simulink model "selector4"  (R2015a)
settings: Solver=FixedStepDiscrete  StartTime=0.0  StopTime=10.0  RelTol=1e-3
settings Model: CovSFcnEnable=off  Creator=arnaud  LastModifiedBy=ktrinh
settings DataIOCC: SaveFormat=StructureWithTime  SignalLoggingSaveFormat=ModelDataLogs
settings OptimizationCC: ExpressionDepthLimit=2147483647
settings DebuggingCC: UnderspecifiedInitializationDetection=Classic  MergeDetectMultiDrivingBlocksExec=none  SolverPrmCheckMsg=warning  FcnCallInpInsideContextMsg=EnableAllAsWarning  StateNameClashWarn=warning
settings GRTTargetCC: CombineOutputUpdateFcns=off  GRTInterface=on

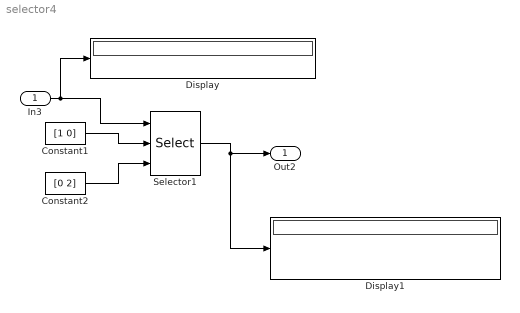
== system selector4 ==
  In3 : Inport  PortDimensions=[2 3]
  Constant1 : Constant  Value=[1 0]
  Constant2 : Constant  Value=[0 2]
  Display : Display
  Display1 : Display
  Selector1 : Selector  NumberOfDimensions=2  IndexMode=Zero-based  InputPortWidth=3  IndexOptions=Index vector (port),Starting and ending indices (port)  Indices=[2 1],1  OutputSizes=1,2
  Out2 : Outport
  wires:
  Constant1/1 -> Selector1/2
  In3/1 -> Display/1, Selector1/1
  Selector1/1 -> Display1/1, Out2/1
  Constant2/1 -> Selector1/3
